simulink model "SG_SinglemotorTest"  (R2022a)
settings: Solver=ode4  StartTime=0.0  StopTime=14  FixedStep=1/(communication_rate*2)  MaxStep=0.001  RelTol=1e-3  AbsTol=1e-3  EnableMultiTasking=on
values from neighbouring files (symbols this model uses):
  communication_rate = 500    [initialization.m]    (also in testScript.m; testState.m)
  dphi_IC = 0    [initialization.m]
  dr_IC = 0    [initialization.m]
  Kd = 5    [testState.m]
  Kd_phi_IC = 0    [initialization.m]
  Kd_r_IC = 0    [initialization.m]
  Kp = 10    [testState.m]
  Kp_phi_IC = 0    [initialization.m]
  Kp_r_IC = 0    [initialization.m]
  phi_IC = 0    [initialization.m]
  r_IC = 0    [initialization.m]
libraries: speedgoatlib_IO691 x4, canmsglib x3, simulink x2
settings Model: Creator=user  LastModifiedBy=Mechatronics
settings SolverCC: AutoScaleAbsTol=off  ConcurrentTasks=on  ZeroCrossAlgorithm=Adaptive  PositivePriorityOrder=on  AutoInsertRateTranBlk=on  MaxZcPerStep=1
settings DataIOCC: LimitDataPoints=on  MaxDataPoints=10000
settings OptimizationCC: BlockReduction=off  OptimizeBlockIOStorage=off
settings DebuggingCC: TasksWithSamePriorityMsg=none  UnconnectedInputMsg=warning  UnconnectedOutputMsg=warning  UnconnectedLineMsg=warning  AllowSymbolicDim=off  SFUnexpectedBacktrackingDiag=warning  SFNoUnconditionalDefaultTransitionDiag=warning  SFExecutionAtInitializationDiag=none  SFMachineParentedDataDiag=warning  ArithmeticOperatorsInVariantConditions=warning
settings HardwareCC: ProdBitPerLong=64  ProdLongLongMode=on  ProdHWDeviceType=Intel->x86-64 (Linux 64)
settings SFSimCC: SimUseLocalCustomCode=off  CustomCodeUndefinedFunction=UseInterfaceOnly
settings RTWCC: Description=Simulink Real-Time  SystemTargetFile=slrealtime.tlc  TemplateMakefile=slrealtime_default_tmf  RTWUseLocalCustomCode=off  Toolchain=Simulink Real-Time Toolchain  BuildConfiguration=Faster Runs  CodeExecutionProfiling=on  TargetLang=C++  DLArmComputeVersion=19.05
settings CodeAppCC: StateflowObjectComments=on
settings ConfigComp: CovMetricSettings=dw  CovSaveCumulativeToWorkspaceVar=on  CovSaveSingleToWorkspaceVar=on  CovExternalEMLEnable=off  CovSFcnEnable=off
settings SimscapeCC: SimscapeLogType=all  SimscapeLogSimulationStatistics=on  SimscapeLogDataHistory=10000
settings ExplorerConfigSet: InternalSimMechanicsExplorerSettings="<ExplorerConfiguration><canonicalview>planar_xy</canonicalview><AnimationSetting><BasePlaybackSpeed>1.0</BasePlaybackSpeed><PlaybackSpeedFactor>0.5</PlaybackSpeedFactor></AnimationSetting><TilePanel><TileInfo><Tiles Columns=\"1\" Count=\"1\" Rows=\"1\"><Column Weight=\"1\"/><Row Weight=\"1\"/><Tile Height=\"1\" Width=\"1\" X=\"0\" Y=\"0\"/></Tiles></TileInfo><SceneInfo><SceneViewer><BGColor><R>0.60000002384185791</R><G>0.60000002384185791</G><B>0.60000002384185791</B></BGColor><Camera><DoPerspective>off</DoPerspective><Position><X>-1.75490981765257059</X><Y>-0.0773030896581384797</Y><Z>0.0348947486595036771</Z></Position><Center><X>0.999999770911101038</X><Y>-0.0773030896581384797</Y><Z>0.0348947486595036771</Z></Center><Up><X>-0</X><Y>1</Y><Z>0</Z></Up><ViewLimDist>1</ViewLimDist><YLim>1.12613649771734692</YLim><XLim>1.72330216917466328</XLim></Camera></SceneViewer></SceneInfo></TilePanel><MechEditorPanel><Cameras/><GfxPanelCameraMap/><VideoCreator><PlaybackSpeedRatio>1.0</PlaybackSpeedRatio><FrameRate>30</FrameRate><VideoFormat>Motion JPEG AVI</VideoFormat><FrameSize>auto</FrameSize></VideoCreator></MechEditorPanel></ExplorerConfiguration>"

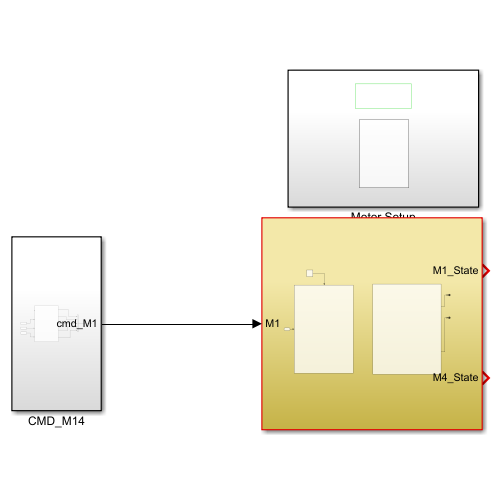
[thumbnail: Simulink's stored preview of the top-level diagram]
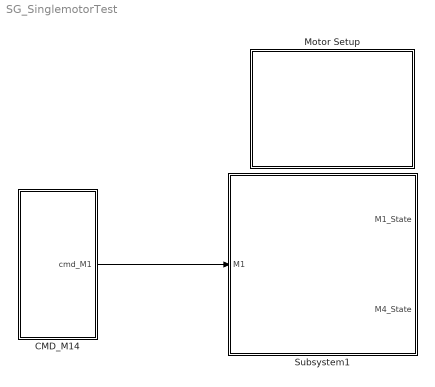
== system SG_SinglemotorTest ==
  CMD_M14 : Subsystem
  Motor Setup : Subsystem
  Subsystem1 : Subsystem
  wires:
  CMD_M14/1(cmd_M1) -> Subsystem1/1(M1)

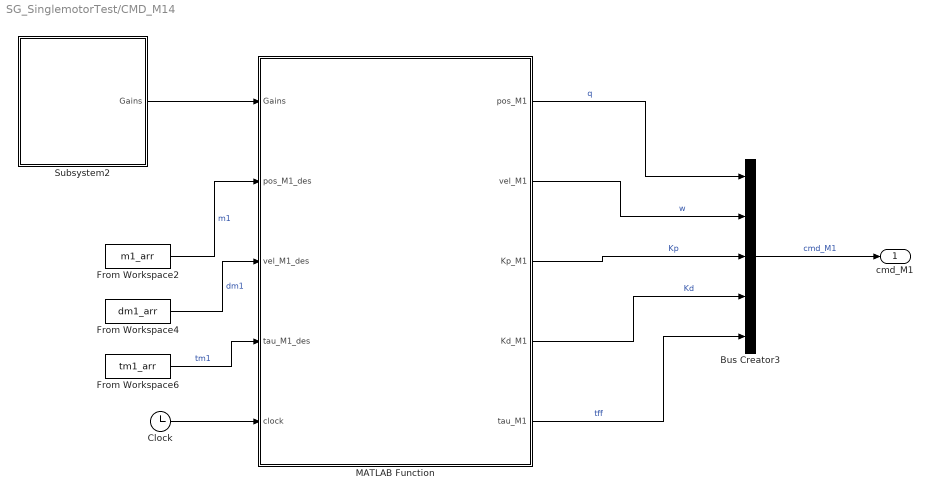
== system SG_SinglemotorTest/CMD_M14 ==
  Bus Creator3 : BusCreator  Inputs=5  OutDataTypeStr=Bus: MotorCmd
  Clock : Clock
  From Workspace2 : FromWorkspace  VariableName=m1_arr  SampleTime=1/communication_rate  Interpolate=off  OutputAfterFinalValue=Cyclic repetition
  From Workspace4 : FromWorkspace  VariableName=dm1_arr  SampleTime=1/communication_rate  Interpolate=off  OutputAfterFinalValue=Cyclic repetition
  From Workspace6 : FromWorkspace  VariableName=tm1_arr  SampleTime=1/communication_rate  Interpolate=off  OutputAfterFinalValue=Cyclic repetition
  MATLAB Function : MATLAB Function  TreatAsAtomicUnit=on
  Subsystem2 : Subsystem
  cmd_M1 : Outport
  wires:
  MATLAB Function/3(Kp_M1) -> Bus Creator3/3  "Kp"
  MATLAB Function/2(vel_M1) -> Bus Creator3/2  "w"
  MATLAB Function/1(pos_M1) -> Bus Creator3/1  "q"
  Bus Creator3/1 -> cmd_M1/1  "cmd_M1"
  MATLAB Function/4(Kd_M1) -> Bus Creator3/4  "Kd"
  MATLAB Function/5(tau_M1) -> Bus Creator3/5  "tff"
  From Workspace4/1 -> MATLAB Function/3(vel_M1_des)  "dm1"
  From Workspace6/1 -> MATLAB Function/4(tau_M1_des)  "tm1"
  From Workspace2/1 -> MATLAB Function/2(pos_M1_des)  "m1"
  Subsystem2/1(Gains) -> MATLAB Function/1(Gains)
  Clock/1 -> MATLAB Function/5(clock)

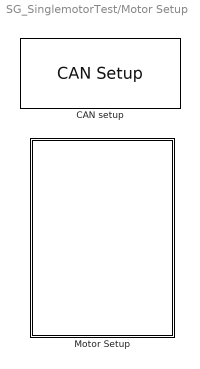
== system SG_SinglemotorTest/Motor Setup ==
  CAN setup : speedgoatlib_IO691/Legacy/CAN Setup   moduletype=IO691  id=1  pciSlot=-1  chn1=CAN (HS)  chn2=CAN (HS)  chn3=Disabled  chn4=Disabled  initStruct=[]  termStruct=[struct('Channel',1,'Protocol','CAN','BRS',0,'Type','Standard','Identifier',3,'Data',[255, 255, 255, 255, 255, 255, 255, 253],'Pause',0.001),struct('Channel',1,'Protocol','CAN','BRS',0,'Type','Standard','Identifier',2,'Data',[255, 255, 255, 255, 255, 255, 255, 253],'Pause',0.001),struct('Channel',2,'Protocol','CAN','BRS',0,'Type','Standard','Identifier',4,'Data',[255, 255, 255, 255, 255, 255, 255, 253],'Pause',0.001), struct('Channel',2,'Protocol','CAN','BRS',0,'Type','Standard','Identifier',1,'Data',[255, 255, 255, 255, 255, 255, 255, 253],'Pause',0.001)]  ArbitrationbdrChn1=1.0 MBaud  ArbitrationManbdrChn1=[2,8,31,8]  FdbdrChn1=1.0 MBaud  FdManbdrChn1=[2,8,31,8]  ArbitrationbdrChn2=1.0 MBaud  ArbitrationManbdrChn2=[2,8,31,8]  FdbdrChn2=1.0 MBaud  FdManbdrChn2=[2,8,31,8]  ArbitrationbdrChn3=1.0 MBaud  ArbitrationManbdrChn3=[2,8,31,8]  FdbdrChn3=5.0 MBaud  FdManbdrChn3=[2,2,5,2]  ArbitrationbdrChn4=1.0 MBaud  ArbitrationManbdrChn4=[2,8,31,8]  FdbdrChn4=5.0 MBaud  FdManbdrChn4=[2,2,5,2]  moduleInitValues=[691 1 -1 -1]
      settings: SourceProductName=Simulink Real-Time: Speedgoat I/O Blockset
  Motor Setup : Subsystem

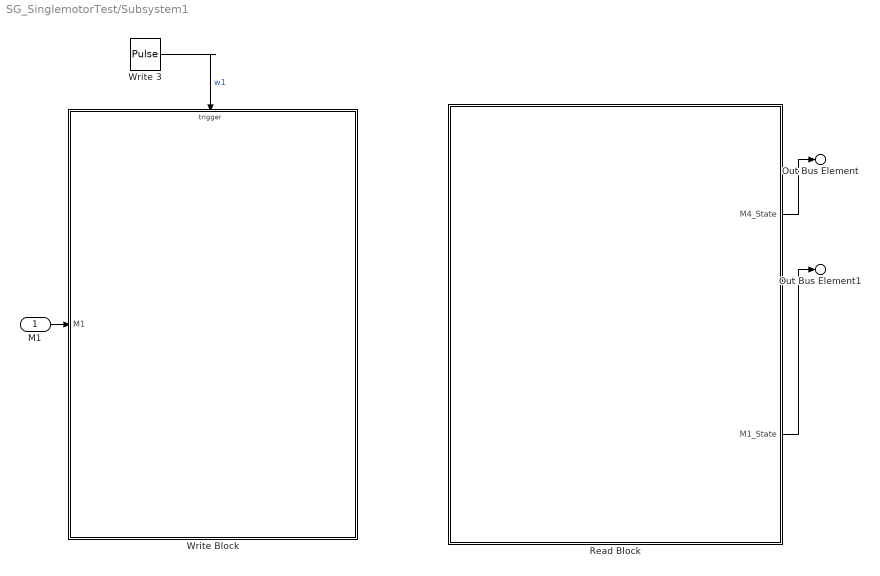
== system SG_SinglemotorTest/Subsystem1 ==
  M1 : Inport
  Read Block : Subsystem
  Write 3 : DiscretePulseGenerator  PulseType=Time based  Period=1/communication_rate  PulseWidth=50  PhaseDelay=3
  Write Block : Subsystem  TreatAsAtomicUnit=on
  Out Bus Element1 : Outport  VectorParamsAs1DForOutWhenUnconnected=off  PortName=M1_State
  Out Bus Element : Outport  Port=2  VectorParamsAs1DForOutWhenUnconnected=off  PortName=M4_State
  wires:
  Write 3/1 -> Write Block/Trigger  "w1"
  M1/1 -> Write Block/1(M1)
  Read Block/1(M4_State) -> Out Bus Element/1
  Read Block/2(M1_State) -> Out Bus Element1/1

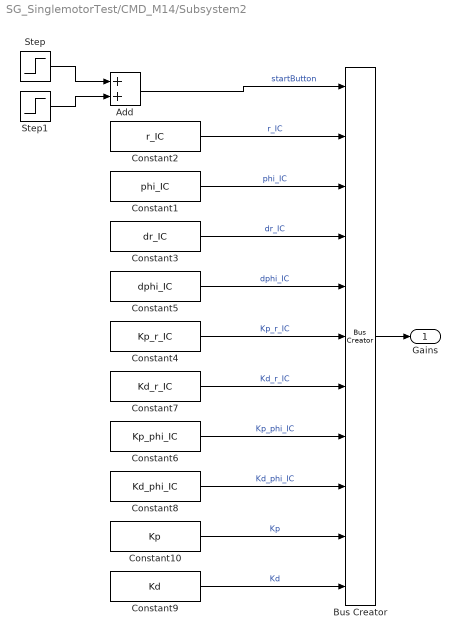
== system SG_SinglemotorTest/CMD_M14/Subsystem2 ==
  Add : Sum
  Bus Creator : BusCreator  Inputs=11  OutDataTypeStr=Bus: Gains
  Constant1 : Constant  Value=phi_IC
  Constant10 : Constant  Value=Kp
  Constant2 : Constant  Value=r_IC
  Constant3 : Constant  Value=dr_IC
  Constant4 : Constant  Value=Kp_r_IC
  Constant5 : Constant  Value=dphi_IC
  Constant6 : Constant  Value=Kp_phi_IC
  Constant7 : Constant  Value=Kd_r_IC
  Constant8 : Constant  Value=Kd_phi_IC
  Constant9 : Constant  Value=Kd
  Step : Step  Time=3  After=0  SampleTime=0
  Step1 : Step  Time=7.5  After=2  SampleTime=0
  Gains : Outport
  wires:
  Step1/1 -> Add/2
  Step/1 -> Add/1
  Constant9/1 -> Bus Creator/11  "Kd"
  Constant10/1 -> Bus Creator/10  "Kp"
  Constant1/1 -> Bus Creator/3  "phi_IC"
  Constant3/1 -> Bus Creator/4  "dr_IC"
  Constant5/1 -> Bus Creator/5  "dphi_IC"
  Constant4/1 -> Bus Creator/6  "Kp_r_IC"
  Constant7/1 -> Bus Creator/7  "Kd_r_IC"
  Constant6/1 -> Bus Creator/8  "Kp_phi_IC"
  Constant8/1 -> Bus Creator/9  "Kd_phi_IC"
  Constant2/1 -> Bus Creator/2  "r_IC"
  Add/1 -> Bus Creator/1  "startButton"
  Bus Creator/1 -> Gains/1

== system SG_SinglemotorTest/Motor Setup/Motor Setup ==
  Back : Subsystem

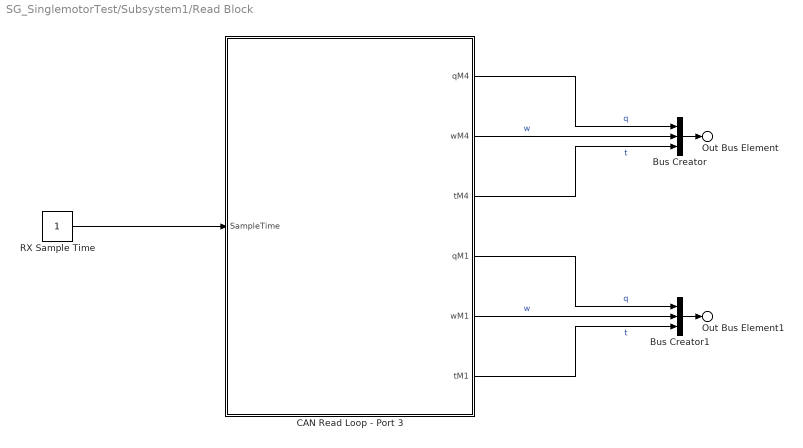
== system SG_SinglemotorTest/Subsystem1/Read Block ==
  Bus Creator : BusCreator  Inputs=3  OutDataTypeStr=Bus: MotorState
  Bus Creator1 : BusCreator  Inputs=3  OutDataTypeStr=Bus: MotorState
  CAN Read Loop - Port 3 : Subsystem  TreatAsAtomicUnit=on
  RX Sample Time : Constant  SampleTime=1/500
  Out Bus Element : Outport  VectorParamsAs1DForOutWhenUnconnected=off  PortName=M4_State
  Out Bus Element1 : Outport  Port=2  VectorParamsAs1DForOutWhenUnconnected=off  PortName=M1_State
  wires:
  RX Sample Time/1 -> CAN Read Loop - Port 3/1(SampleTime)
  CAN Read Loop - Port 3/3(tM4) -> Bus Creator/3  "t"
  CAN Read Loop - Port 3/2(wM4) -> Bus Creator/2  "w"
  Bus Creator1/1 -> Out Bus Element1/1
  CAN Read Loop - Port 3/6(tM1) -> Bus Creator1/3  "t"
  CAN Read Loop - Port 3/1(qM4) -> Bus Creator/1  "q"
  CAN Read Loop - Port 3/5(wM1) -> Bus Creator1/2  "w"
  Bus Creator/1 -> Out Bus Element/1
  CAN Read Loop - Port 3/4(qM1) -> Bus Creator1/1  "q"

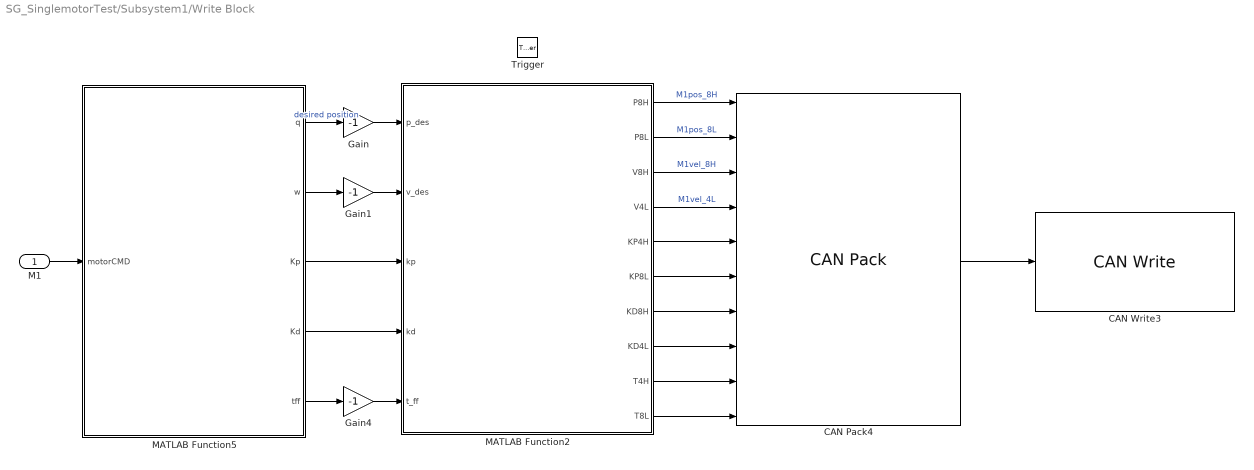
== system SG_SinglemotorTest/Subsystem1/Write Block ==
  M1 : Inport
  Trigger : TriggerPort  VariantControl=Variant
  CAN Pack4 : canmsglib/CAN Pack  MsgList=(none)  MsgName=MotorControl  MsgIDType=Standard (11-bit identifier)  MsgIdentifier=1  MsgLength=8  Remote=off  ApplyMinMax=off  BusOutput=off  SignalInfo={ 'Motor postition 8-H', '0', '8', 'LE', 'unsigned', 'Standard', '0', '1', '0', '-Inf', 'Inf'; 'Motor position 8-L', '8', '8', 'LE', 'unsigned', 'Standard', '0', '1', '0', '-Inf', 'Inf'; 'Motor speed 8-H', '16', '8', 'LE', 'unsigned', 'Standard', '0', '1', '0', '-Inf', 'Inf'; 'Motor speed 4-L', '28', '4', 'LE', 'unsigned', 'Standard', '0', '1', '0', '-Inf', 'Inf'; 'KP 4-H', '24', '4', 'LE', 'unsigned', 'Standard', '0', '1', '0', '-Inf', 'Inf'; 'KP 8-L', '32', '8', 'LE', 'unsigned', 'Standard', '0', '1', '0', '-Inf', 'Inf'; 'KD 8-H', '40', '8', 'LE', 'unsigned', 'Standard', '0', '1', '0', '-Inf', 'Inf'; 'KD 4-L', '52', '4', 'LE', 'unsigned', 'Standard', '0', '1', '0', '-Inf', 'Inf'; 'Current 4-H', '48', '4', 'LE', 'unsigned', 'Standard', '0', '1', '0', '-Inf', 'Inf'; 'Current 8-L', '56', '8', 'LE', 'unsigned', 'Standard', '0', '1', '0', '-Inf', 'Inf' }
      settings: SourceProductBaseCode=XP,ME,VN  DataFormat=manually specified signals
  CAN Write3 : speedgoatlib_IO691/Legacy/CAN Write  id=1  ts=-1  channel=2  messageType=CAN  BusInput=off  enableStatusPort=off  canType=CAN (HS)  initValues=[691 1 -1 1 1 1 0 0]
      settings: SourceProductName=Simulink Real-Time: Speedgoat Library
  Gain : Gain  Gain=-1
  Gain1 : Gain  Gain=-1
  Gain4 : Gain  Gain=-1
  MATLAB Function2 : MATLAB Function  TreatAsAtomicUnit=on
  MATLAB Function5 : MATLAB Function  TreatAsAtomicUnit=on
  wires:
  MATLAB Function2/8(KD4L) -> CAN Pack4/8
  Gain4/1 -> MATLAB Function2/5(t_ff)
  MATLAB Function2/7(KD8H) -> CAN Pack4/7
  MATLAB Function2/2(P8L) -> CAN Pack4/2  "M1pos_8L"
  MATLAB Function2/10(T8L) -> CAN Pack4/10
  CAN Pack4/1 -> CAN Write3/1
  MATLAB Function2/3(V8H) -> CAN Pack4/3  "M1vel_8H"
  MATLAB Function5/4(Kd) -> MATLAB Function2/4(kd)
  MATLAB Function2/1(P8H) -> CAN Pack4/1  "M1pos_8H"
  MATLAB Function2/6(KP8L) -> CAN Pack4/6
  MATLAB Function5/5(tff) -> Gain4/1
  MATLAB Function5/1(q) -> Gain/1  "desired position"
  MATLAB Function2/9(T4H) -> CAN Pack4/9
  Gain/1 -> MATLAB Function2/1(p_des)
  MATLAB Function2/4(V4L) -> CAN Pack4/4  "M1vel_4L"
  Gain1/1 -> MATLAB Function2/2(v_des)
  MATLAB Function2/5(KP4H) -> CAN Pack4/5
  MATLAB Function5/2(w) -> Gain1/1
  MATLAB Function5/3(Kp) -> MATLAB Function2/3(kp)
  M1/1 -> MATLAB Function5/1(motorCMD)

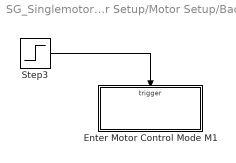
== system SG_SinglemotorTest/Motor Setup/Motor Setup/Back ==
  Enter Motor Control Mode M1 : Subsystem  TreatAsAtomicUnit=on
  Step3 : Step
  wires:
  Step3/1 -> Enter Motor Control Mode M1/Trigger

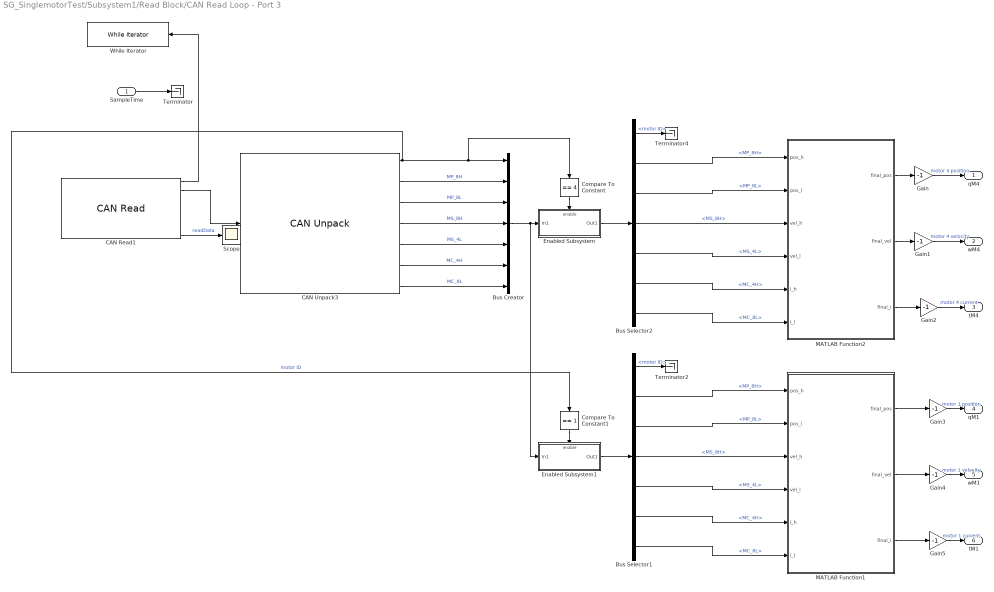
== system SG_SinglemotorTest/Subsystem1/Read Block/CAN Read Loop - Port 3 ==
  SampleTime : Inport
  Bus Creator : BusCreator  Inputs=7
  Bus Selector1 : BusSelector  OutputSignals=motor ID,MP_8H,MP_8L,MS_8H,MS_4L,MC_4H,MC_8L
  Bus Selector2 : BusSelector  OutputSignals=motor ID,MP_8H,MP_8L,MS_8H,MS_4L,MC_4H,MC_8L
  CAN Read1 : speedgoatlib_IO691/Legacy/CAN Read  id=1  ts=-1  channel=2  messageType=CAN + RAW  canType=CAN (HS)  BusOutput=off  initValues=[691 1 -1 1 3 1 0]
      settings: SourceProductName=Simulink Real-Time: Speedgoat Library
  CAN Unpack3 : canmsglib/CAN Unpack  MsgList=(none)  MsgName=CAN Msg  MsgIDType=Standard (11-bit identifier)  MsgIdentifier=0  MsgLength=8  SignalInfo={ 'Drive ID', '0', '8', 'LE', 'unsigned', 'Standard', '0', '1', '0', '-Inf', 'Inf'; 'Motor position 8-H', '8', '8', 'LE', 'unsigned', 'Standard', '0', '1', '0', '-Inf', 'Inf'; 'Motor position 8-L', '16', '8', 'LE', 'unsigned', 'Standard', '0', '1', '0', '-Inf', 'Inf'; 'Motor speed 8-H', '24', '8', 'LE', 'unsigned', 'Standard', '0', '1', '0', '-Inf', 'Inf'; 'Motor speed 4-L', '36', '4', 'LE', 'unsigned', 'Standard', '0', '1', '0', '-Inf', 'Inf'; 'Current 4-H', '32', '4', 'LE', 'unsigned', 'Standard', '0', '1', '0', '-Inf', 'Inf'; 'Current 8-L', '40', '8', 'LE', 'unsigned', 'Standard', '0', '1', '0', '-Inf', 'Inf' }  IDPort=off  TimestampPort=off  ErrorPort=off  RemotePort=off  LengthPort=off  StatusPort=off  ApplyMinMax=off
      settings: SourceProductBaseCode=XP,ME,VN
  Compare To Constant : simulink/Logic and Bit Operations/Compare To Constant  relop===  const=4  OutDataTypeStr=boolean
  Compare To Constant1 : simulink/Logic and Bit Operations/Compare To Constant  relop===  const=1  OutDataTypeStr=boolean
  Enabled Subsystem : Subsystem  TreatAsAtomicUnit=on
  Enabled Subsystem1 : Subsystem  TreatAsAtomicUnit=on
  Gain{,1..5} (6 alike) : Gain  Gain=-1
  MATLAB Function1 : MATLAB Function  TreatAsAtomicUnit=on
  MATLAB Function2 : MATLAB Function  TreatAsAtomicUnit=on
  Scope : Scope
  Terminator : Terminator
  Terminator2 : Terminator
  Terminator4 : Terminator
  While Iterator : WhileIterator  MaxIters=501  WhileBlockType=do-while
  qM4 : Outport
  wM4 : Outport  Port=2
  tM4 : Outport  Port=3
  qM1 : Outport  Port=4
  wM1 : Outport  Port=5
  tM1 : Outport  Port=6
  wires:
  SampleTime/1 -> Terminator/1
  CAN Read1/1 -> While Iterator/1
  Bus Selector2/1 -> Terminator4/1  "<motor ID>"
  Bus Selector1/4 -> MATLAB Function1/3(vel_h)  "<MS_8H>"
  CAN Unpack3/7 -> Bus Creator/7  "MC_8L"
  CAN Unpack3/3 -> Bus Creator/3  "MP_8L"
  Gain3/1 -> qM1/1  "motor 1 position"
  Gain5/1 -> tM1/1  "motor 1 current"
  Gain1/1 -> wM4/1  "motor 4 velocity"
  Gain/1 -> qM4/1  "motor 4 position"
  CAN Read1/2 -> CAN Unpack3/1
  MATLAB Function1/1(final_pos) -> Gain3/1
  MATLAB Function2/2(final_vel) -> Gain1/1
  Gain2/1 -> tM4/1  "motor 4 current"
  Bus Selector1/7 -> MATLAB Function1/6(i_l)  "<MC_8L>"
  Bus Selector1/5 -> MATLAB Function1/4(vel_l)  "<MS_4L>"
  MATLAB Function1/2(final_vel) -> Gain4/1
  Bus Selector1/1 -> Terminator2/1  "<motor ID>"
  Bus Creator/1 -> Enabled Subsystem1/1(In1), Enabled Subsystem/1(In1)
  Bus Selector1/2 -> MATLAB Function1/1(pos_h)  "<MP_8H>"
  Bus Selector1/6 -> MATLAB Function1/5(i_h)  "<MC_4H>"
  CAN Unpack3/4 -> Bus Creator/4  "MS_8H"
  CAN Unpack3/5 -> Bus Creator/5  "MS_4L"
  Bus Selector2/4 -> MATLAB Function2/3(vel_h)  "<MS_8H>"
  Enabled Subsystem/1(Out1) -> Bus Selector2/1
  Bus Selector2/6 -> MATLAB Function2/5(i_h)  "<MC_4H>"
  Bus Selector1/3 -> MATLAB Function1/2(pos_l)  "<MP_8L>"
  Bus Selector2/7 -> MATLAB Function2/6(i_l)  "<MC_8L>"
  CAN Unpack3/1 -> Bus Creator/1, Compare To Constant/1, Compare To Constant1/1  "motor ID"
  Enabled Subsystem1/1(Out1) -> Bus Selector1/1
  Compare To Constant/1 -> Enabled Subsystem/Enable
  Bus Selector2/3 -> MATLAB Function2/2(pos_l)  "<MP_8L>"
  Bus Selector2/2 -> MATLAB Function2/1(pos_h)  "<MP_8H>"
  CAN Unpack3/6 -> Bus Creator/6  "MC_4H"
  MATLAB Function2/3(final_i) -> Gain2/1
  Gain4/1 -> wM1/1  "motor 1 velocity"
  Compare To Constant1/1 -> Enabled Subsystem1/Enable
  Bus Selector2/5 -> MATLAB Function2/4(vel_l)  "<MS_4L>"
  MATLAB Function2/1(final_pos) -> Gain/1
  CAN Unpack3/2 -> Bus Creator/2  "MP_8H"
  MATLAB Function1/3(final_i) -> Gain5/1
  CAN Read1/7 -> Scope/1  "readData"

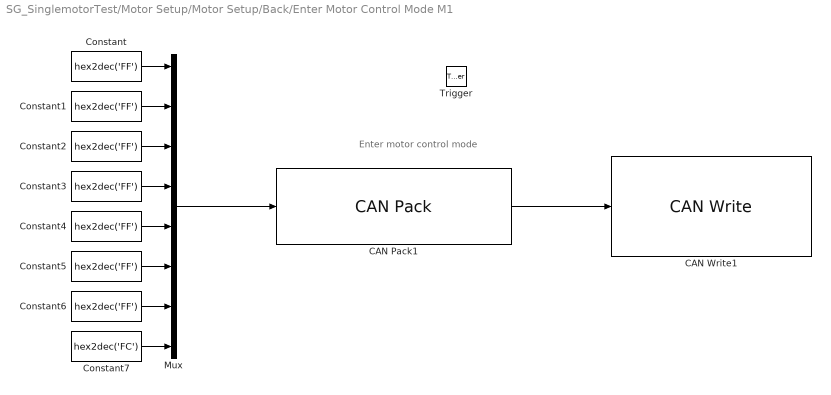
== system SG_SinglemotorTest/Motor Setup/Motor Setup/Back/Enter Motor Control Mode M1 ==
  note: Enter motor control mode
  Trigger : TriggerPort  VariantControl=Variant
  CAN Pack1 : canmsglib/CAN Pack  MsgList=(none)  MsgName=CAN Msg  MsgIDType=Standard (11-bit identifier)  MsgIdentifier=1  MsgLength=8  Remote=off  ApplyMinMax=off  BusOutput=off  SignalInfo={ 'Motor postition 8-H', '0', '8', 'LE', 'unsigned', 'Standard', '0', '1', '0', '-Inf', 'Inf'; 'Motor position 8-L', '8', '8', 'LE', 'unsigned', 'Standard', '0', '1', '0', '-Inf', 'Inf'; 'Motor seed 8-H', '16', '8', 'LE', 'unsigned', 'Standard', '0', '1', '0', '-Inf', 'Inf'; 'Motor speed 4-L', '28', '4', 'LE', 'unsigned', 'Standard', '0', '1', '0', '-Inf', 'Inf'; 'KP 4-H', '24', '4', 'LE', 'unsigned', 'Standard', '0', '1', '0', '-Inf', 'Inf'; 'KP 8-L', '32', '8', 'LE', 'unsigned', 'Standard', '0', '1', '0', '-Inf', 'Inf'; 'KP 8-H', '40', '8', 'LE', 'unsigned', 'Standard', '0', '1', '0', '-Inf', 'Inf'; 'KD 4-L', '52', '4', 'LE', 'unsigned', 'Standard', '0', '1', '0', '-Inf', 'Inf'; 'Current 4-H', '48', '4', 'LE', 'unsigned', 'Standard', '0', '1', '0', '-Inf', 'Inf'; 'Current 8-L', '56', '8', 'LE', 'unsigned', 'Standard', '0', '1', '0', '-Inf', 'Inf' }
      settings: SourceProductBaseCode=XP,ME,VN  DataFormat=raw data
  CAN Write1 : speedgoatlib_IO691/Legacy/CAN Write  id=1  ts=-1  channel=2  messageType=CAN  BusInput=off  enableStatusPort=off  canType=CAN (HS)  initValues=[691 1 -1 1 1 1 0 0]
      settings: SourceProductName=Simulink Real-Time: Speedgoat Library
  Constant{,1..6} (7 alike) : Constant  Value=hex2dec('FF')  OutDataTypeStr=uint8  SampleTime=-1
  Constant7 : Constant  Value=hex2dec('FC')  OutDataTypeStr=uint8  SampleTime=-1
  Mux : Mux  Inputs=8
  wires:
  CAN Pack1/1 -> CAN Write1/1
  Mux/1 -> CAN Pack1/1
  Constant7/1 -> Mux/8
  Constant4/1 -> Mux/5
  Constant1/1 -> Mux/2
  Constant5/1 -> Mux/6
  Constant3/1 -> Mux/4
  Constant2/1 -> Mux/3
  Constant/1 -> Mux/1
  Constant6/1 -> Mux/7

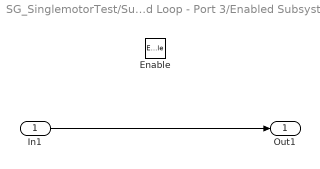
== system SG_SinglemotorTest/Subsystem1/Read Block/CAN Read Loop - Port 3/Enabled Subsystem ==
  In1 : Inport
  Enable : EnablePort
  Out1 : Outport
  wires:
  In1/1 -> Out1/1

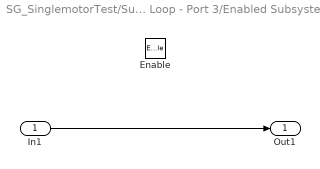
== system SG_SinglemotorTest/Subsystem1/Read Block/CAN Read Loop - Port 3/Enabled Subsystem1 ==
  In1 : Inport
  Enable : EnablePort
  Out1 : Outport
  wires:
  In1/1 -> Out1/1

== matlab function SG_SinglemotorTest/Subsystem1/Write Block/MATLAB Function2 ==
  data: p_des input; P8H output; v_des input; kp input; kd input; t_ff input; P8L output; V8H output; V4L output; KP4H output; KP8L output; KD8H output; KD4L output; T4H output; T8L output
function [P8H,P8L,V8H,V4L,KP4H,KP8L,KD8H,KD4L,T4H,T8L] = AK1090(p_des, v_des, kp, kd, t_ff)
    % Coppied from AK70-10 manual
    % NB: CONSTANTS FOR AK70-10
    p_min = -12.5; % rad
    p_max = +12.5; % rad
    v_min = -50.0; % rad/s
    v_max = +50.0; % rad/s
    t_min = -65.0; % Nm
    t_max = +65.0; % Nm
    kp_min = 0;
    kp_max = 500;
    kd_min = 0;
    kd_max = 5;
    
    % bound inputs
    p_des = min([max([p_min,p_des]),p_max]);
    v_des = min([max([v_min,v_des]),v_max]);
    kp = min([max([kp_min,kp]),kp_max]);
    kd = min([max([kd_min,kd]),kd_max]);
    t_ff = min([max([t_min,t_ff]),t_max]);
    
    % convert floats to unsigned integers
    p_int = float_to_uint(p_des, p_min, p_max, 16);
    v_int = float_to_uint(v_des, v_min, v_max, 12);
    kp_int = float_to_uint(kp, kp_min, kp_max, 12);
    kd_int = float_to_uint(kd, kd_min, kd_max, 12);
    t_int = float_to_uint(t_ff, t_min, t_max, 12);
    
    % break up for CAN frame 
    P8H = bitshift(p_int, -8); % 8 higher bits
    P8L = bitand(p_int, 0xFF); % 8 lower bits
    V8H = bitshift(v_int, -4); % 8 higher bits
    V4L = bitand(v_int, 0xF); % 4 lower bits
    KP4H = bitshift(kp_int, -8); % 4 higher bits
    KP8L = bitand(kp_int, 0xFF); % 8 lower bits
    KD8H = bitshift(kd_int, -4); % 8 higher bits
    KD4L = bitand(kd_int, 0xF); % 4 lower bits
    T4H = bitshift(t_int, -8); % 4 higher bits
    T8L = bitand(t_int, 0xFF); % 8 lower bits
    
    % Converts a float to an unsigned int, given range and number of bits
    function x_int = float_to_uint(x, x_min, x_max, n_bits)
        span = x_max - x_min;
        min([max([x_min,x]),x_max])
        x_int = ((x - x_min)*(bitshift(1, n_bits) / span));
    end
end
%final_values = desired_pos,desired_vel,desired_kp,desired_kd,desired_tau;

== matlab function SG_SinglemotorTest/Subsystem1/Read Block/CAN Read Loop - Port 3/MATLAB Function1 ==
  data: pos_h input; final_pos output; pos_l input; vel_h input; vel_l input; i_h input; i_l input; final_vel output; final_i output
function [final_pos,final_vel,final_i] = fcn(pos_h,pos_l,vel_h,vel_l,i_h,i_l)
% ------------------------------------
max_pos = 12.5;
min_pos = -12.5;
span_pos = max_pos - min_pos;
offset_pos = max_pos;

pos = bitshift(pos_h,8);
combined_pos = bitor(pos,pos_l);

range_pos = ((combined_pos*span_pos)/(2^16-1))-offset_pos;

final_pos = (range_pos*4*pi)/12.5;
% ------------------------------------
max_vel = 23.24;
min_vel = -23.24;
span_vel = max_vel - min_vel;
offset_vel = max_vel;
vel = bitshift(vel_h,4);
combined_vel = bitor(vel,vel_l);

final_vel = ((combined_vel*span_vel)/(2^12-1))-offset_vel;

% ------------------------------------
max_i = 54;
min_i = -54;
span_i = max_i - min_i;
offset_i = max_i;
i = bitshift(i_h,8);
combined_i = bitor(i,i_l);

final_i = ((combined_i*span_i)/(2^12-1))-offset_i;
end

== matlab function SG_SinglemotorTest/Subsystem1/Read Block/CAN Read Loop - Port 3/MATLAB Function2 ==
  data: pos_h input; final_pos output; pos_l input; vel_h input; vel_l input; i_h input; i_l input; final_vel output; final_i output
function [final_pos,final_vel,final_i] = fcn(pos_h,pos_l,vel_h,vel_l,i_h,i_l)
% ------------------------------------
max_pos = 12.5;
min_pos = -12.5;
span_pos = max_pos - min_pos;
offset_pos = max_pos;

pos = bitshift(pos_h,8);
combined_pos = bitor(pos,pos_l);

range_pos = ((combined_pos*span_pos)/(2^16-1))-offset_pos;

final_pos = (range_pos*4*pi)/12.5;
% ------------------------------------
max_vel = 50;
min_vel = -50;
span_vel = max_vel - min_vel;
offset_vel = max_vel;
vel = bitshift(vel_h,4);
combined_vel = bitor(vel,vel_l);

final_vel = ((combined_vel*span_vel)/(2^12-1))-offset_vel;

% ------------------------------------
max_i = 65;
min_i = -65;
span_i = max_i - min_i;
offset_i = max_i;
i = bitshift(i_h,8);
combined_i = bitor(i,i_l);

final_i = ((combined_i*span_i)/(2^12-1))-offset_i;
end

== matlab function SG_SinglemotorTest/Subsystem1/Write Block/MATLAB Function5 ==
  data: motorCMD input; q output; w output; Kp output; Kd output; tff output
function [q,w,Kp,Kd,tff] = cmd(motorCMD)

    q = motorCMD.q;
    w = motorCMD.w;
    Kp = motorCMD.Kp;
    Kd = motorCMD.Kd;
    tff = motorCMD.tff;

end

== matlab function SG_SinglemotorTest/CMD_M14/MATLAB Function ==
  data: Gains input; pos_M1_des input; vel_M1_des input; tau_M1_des input; pos_M1 output; vel_M1 output; Kp_M1 output; Kd_M1 output; tau_M1 output; clock input
function [pos_M1,vel_M1,Kp_M1,Kd_M1,tau_M1] = dataSelection(Gains,pos_M1_des,vel_M1_des,tau_M1_des,clock)

    if clock>6.2

        pos_M1 = pos_M1_des;

        vel_M1 = vel_M1_des;

        tau_M1 = tau_M1_des;
        Kp_M1 = Gains.Kp;
        Kd_M1 = Gains.Kd;

    else

        pos_M1 = 0;
        vel_M1 = 0;
        tau_M1 = 0;
        Kp_M1 = 0;
        Kd_M1 = 0;
    end
end
